simulink model "pro_3"  (R2020a)
settings: Solver=VariableStepAuto  StartTime=0.0  StopTime=120  RelTol=1e-3
model workspace (MAT data in the model file):
  b = Simulink.Parameter
  b.Value = 50
  b.DataType = 'auto'
  b.Dimensions = [1 1]
  ki = Simulink.Parameter
  ki.Value = 50
  ki.DataType = 'auto'
  ki.Dimensions = [1 1]
  kp = Simulink.Parameter
  kp.Value = 100
  kp.DataType = 'auto'
  kp.Dimensions = [1 1]
  m = Simulink.Parameter
  m.Value = 1000
  m.DataType = 'auto'
  m.Dimensions = [1 1]
  u = Simulink.Parameter
  u.Value = 500
  u.DataType = 'auto'
  u.Dimensions = [1 1]
settings Model: OrderedModelArguments=off  Creator=akhil singh  LastModifiedBy=akhil singh

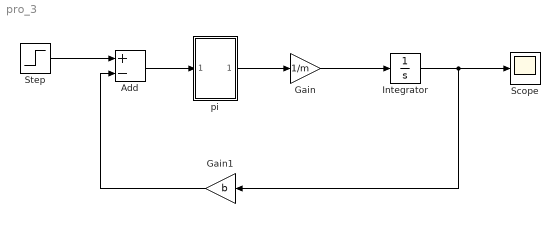
== system pro_3 ==
  Add : Sum  Inputs=+-
  Gain : Gain  Gain=1/m
  Gain1 : Gain  Gain=b
  Integrator : Integrator
  Scope : Scope
  Step : Step  Time=0  After=u  SampleTime=0
  pi : Subsystem
  wires:
  Gain/1 -> Integrator/1
  Step/1 -> Add/1
  Gain1/1 -> Add/2
  Integrator/1 -> Gain1/1, Scope/1
  Add/1 -> pi/1(In1)
  pi/1(Out1) -> Gain/1

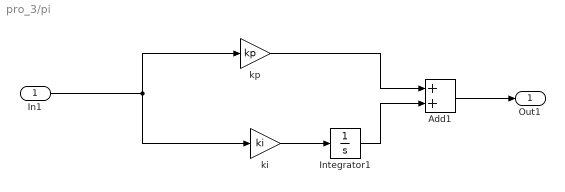
== system pro_3/pi ==
  In1 : Inport
  Add1 : Sum
  Integrator1 : Integrator
  ki : Gain  Gain=ki
  kp : Gain  Gain=kp
  Out1 : Outport
  wires:
  Integrator1/1 -> Add1/2
  In1/1 -> kp/1, ki/1
  ki/1 -> Integrator1/1
  kp/1 -> Add1/1
  Add1/1 -> Out1/1
